simulink model "ffttest"  (Simulink 6.2)
settings: Solver=ode45  StartTime=0.0  StopTime=10.0  RelTol=1e-3
libraries: xbsIndex_r3 x4, fft_library x1
settings Model: LastModifiedBy=mdexter
settings DebuggingCC: SolverPrmCheckMsg=warning

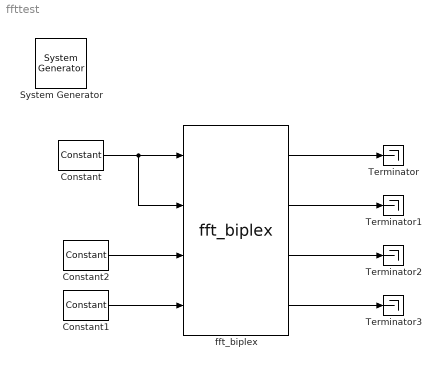
== system ffttest ==
  " System Generator" : xbsIndex_r3/ System Generator  Tag=genX  xilinxfamily=Virtex2  part=xc2v1000  speed=-4  package=bg575  synthesis_tool=XST  directory=./netlist  testbench=off  simulink_period=1  sysclk_period=100  incr_netlist=off  trim_vbits=Everywhere in SubSystem  dbl_ovrd=According to Block Masks  core_generation=According to Block Masks  run_coregen=off  deprecated_control=off  eval_field=0
      settings: AttributesFormatString=System\nGenerator
  Constant : xbsIndex_r3/Constant  const=0  equ=P=C  arith_type=Unsigned  n_bits=36  bin_pt=0  opselect=C  inp2=PCIN>>17  opr=+  inp1=P  carry=CIN  iostate=0  explicit_period=on  period=1  dbl_ovrd=off
  Constant1 : xbsIndex_r3/Constant  const=0  equ=P=C  arith_type=Unsigned  n_bits=10  bin_pt=0  opselect=C  inp2=PCIN>>17  opr=+  inp1=P  carry=CIN  iostate=0  explicit_period=on  period=1  dbl_ovrd=off
  Constant2 : xbsIndex_r3/Constant  const=0  equ=P=C  arith_type=Boolean  n_bits=18  bin_pt=0  opselect=C  inp2=PCIN>>17  opr=+  inp1=P  carry=CIN  iostate=0  explicit_period=on  period=1  dbl_ovrd=off
  Terminator{,1..3} (4 alike) : Terminator
  fft_biplex : fft_library/fft_biplex  FFTSize=10  BitWidth=18  quantization="Round  (unbiased: Even Values)"  overflow=Wrap  add_latency=1  mult_latency=1  bram_latency=1
      link override biplex_core/fft_stage_1/sync_delay_x/Constant: equ=P=C
      link override biplex_core/fft_stage_1/sync_delay_x/Constant1: equ=P=C
      link override biplex_core/fft_stage_1/sync_delay_x/Constant2: equ=P=C
      link override biplex_core/fft_stage_1/sync_delay_x/Constant3: equ=P=C
      link override biplex_core/fft_stage_2/sync_delay_x/Constant: equ=P=C
      link override biplex_core/fft_stage_2/sync_delay_x/Constant1: equ=P=C
      link override biplex_core/fft_stage_2/sync_delay_x/Constant2: equ=P=C
      link override biplex_core/fft_stage_2/sync_delay_x/Constant3: equ=P=C
      link override biplex_cplx_unscrambler/reorder/sync_delay/Constant: equ=P=C
      link override biplex_cplx_unscrambler/reorder/sync_delay/Constant1: equ=P=C
      link override biplex_cplx_unscrambler/reorder/sync_delay/Constant2: equ=P=C
      link override biplex_cplx_unscrambler/reorder/sync_delay/Constant3: equ=P=C
      link override biplex_cplx_unscrambler/reorder1/sync_delay/Constant: equ=P=C
      link override biplex_cplx_unscrambler/reorder1/sync_delay/Constant1: equ=P=C
      link override biplex_cplx_unscrambler/reorder1/sync_delay/Constant2: equ=P=C
      link override biplex_cplx_unscrambler/reorder1/sync_delay/Constant3: equ=P=C
  wires:
  Constant/1 -> fft_biplex/2, fft_biplex/1
  Constant1/1 -> fft_biplex/4
  Constant2/1 -> fft_biplex/3
  fft_biplex/1 -> Terminator/1
  fft_biplex/2 -> Terminator1/1
  fft_biplex/3 -> Terminator2/1
  fft_biplex/4 -> Terminator3/1
